simulink model "PIMPID"  (R2013b)
settings: Solver=FixedStepDiscrete  SolverMode=SingleTasking  StartTime=0.0  StopTime=100  FixedStep=0.1  RelTol=1e-3
libraries: xbsIndex_r4 x23, simulink x1
settings Model: Creator=laca  LastModifiedBy=laca

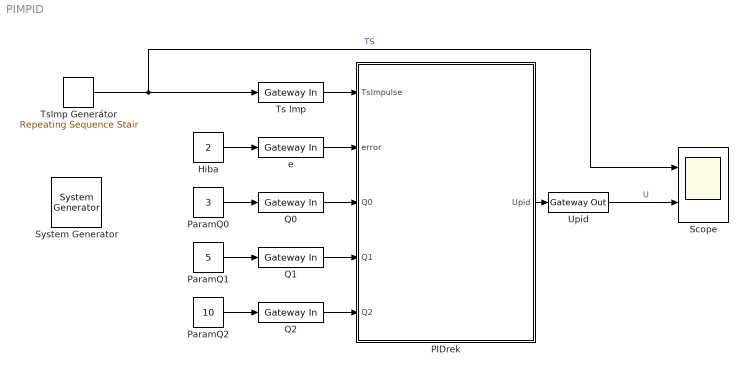
== system PIMPID ==
  " System Generator" : xbsIndex_r4/ System Generator  Tag=genX  xilinxfamily=spartan3e  part=xc3s500e  speed=-4  package=pq208  synthesis_tool=XST  clock_wrapper=Clock Enables  directory=./netlist  proj_type=Project Navigator  Synth_file=XST Defaults  Impl_file=ISE Defaults  testbench=off  simulink_period=1  sysclk_period=20  dcm_input_clock_period=10  incr_netlist=off  trim_vbits=Everywhere in SubSystem  dbl_ovrd=According to Block Masks  core_generation=According to Block Masks  run_coregen=off  deprecated_control=off  eval_field=0  block_type=sysgen
  Hiba : Constant  Value=2
  PIDrek : Subsystem
  ParamQ0 : Constant  Value=3
  ParamQ1 : Constant  Value=5
  ParamQ2 : Constant  Value=10
  Q0 : xbsIndex_r4/Gateway In  gui_display_data_type=Fixed-point  arith_type="Signed  (2's comp)"  n_bits=16  bin_pt=0  preci_type=Single  exp_width=8  frac_width=24  quantization="Round  (unbiased: +/- Inf)"  overflow=Saturate  period=1  dbl_ovrd=off  timing_constraint=None  locs_specified=off  LOCs={}  UseAsADC=off  ADCChannel='1'  inherit_from_input=off  hdl_port=on  block_type=gatewayin
  Q1 : xbsIndex_r4/Gateway In  gui_display_data_type=Fixed-point  arith_type="Signed  (2's comp)"  n_bits=16  bin_pt=0  preci_type=Single  exp_width=8  frac_width=24  quantization="Round  (unbiased: +/- Inf)"  overflow=Saturate  period=1  dbl_ovrd=off  timing_constraint=None  locs_specified=off  LOCs={}  UseAsADC=off  ADCChannel='1'  inherit_from_input=off  hdl_port=on  block_type=gatewayin
  Q2 : xbsIndex_r4/Gateway In  gui_display_data_type=Fixed-point  arith_type="Signed  (2's comp)"  n_bits=16  bin_pt=0  preci_type=Single  exp_width=8  frac_width=24  quantization="Round  (unbiased: +/- Inf)"  overflow=Saturate  period=1  dbl_ovrd=off  timing_constraint=None  locs_specified=off  LOCs={}  UseAsADC=off  ADCChannel='1'  inherit_from_input=off  hdl_port=on  block_type=gatewayin
  Scope : Scope  NumInputPorts=2
      settings: TimeRange=100  YMin=0~-5  YMax=1~5  SaveName=SC
  Ts Imp : xbsIndex_r4/Gateway In  gui_display_data_type=Boolean  arith_type=Boolean  n_bits=16  bin_pt=14  preci_type=Single  exp_width=8  frac_width=24  quantization="Round  (unbiased: +/- Inf)"  overflow=Saturate  period=1  dbl_ovrd=off  timing_constraint=None  locs_specified=off  LOCs={}  UseAsADC=off  ADCChannel='1'  inherit_from_input=off  hdl_port=on  block_type=gatewayin
  TsImp Generátor : simulink/Sources/Repeating Sequence Stair  OutValues="[0 0 1  0 0 0 0 0 0 0 0 0 0 0 0 0 0 0 0 0 ].'"  tsamp=1  OutMin=[]  OutMax=[]  OutDataTypeStr=fixdt('boolean')  OutputDataTypeScalingMode=Specify via dialog  OutDataType=fixdt('boolean')  ConRadixGroup=Best Precision: Vector-wise  OutScaling=[]
  Upid : xbsIndex_r4/Gateway Out  inherit_from_input=off  hdl_port=on  timing_constraint=None  locs_specified=off  LOCs={}  UseAsDAC=off  DACChannel='1'  block_type=gatewayout
  e : xbsIndex_r4/Gateway In  gui_display_data_type=Fixed-point  arith_type="Signed  (2's comp)"  n_bits=16  bin_pt=0  preci_type=Single  exp_width=8  frac_width=24  quantization="Round  (unbiased: +/- Inf)"  overflow=Saturate  period=1  dbl_ovrd=off  timing_constraint=None  locs_specified=off  LOCs={}  UseAsADC=off  ADCChannel='1'  inherit_from_input=off  hdl_port=on  block_type=gatewayin
  wires:
  Ts Imp/1 -> PIDrek/1(TsImpulse)
  Hiba/1 -> e/1
  ParamQ0/1 -> Q0/1
  ParamQ1/1 -> Q1/1
  ParamQ2/1 -> Q2/1
  Upid/1 -> Scope/2  "U"
  TsImp Generátor/1 -> Scope/1, Ts Imp/1  "TS"
  PIDrek/1(Upid) -> Upid/1
  e/1 -> PIDrek/2(error)
  Q0/1 -> PIDrek/3(Q0)
  Q1/1 -> PIDrek/4(Q1)
  Q2/1 -> PIDrek/5(Q2)

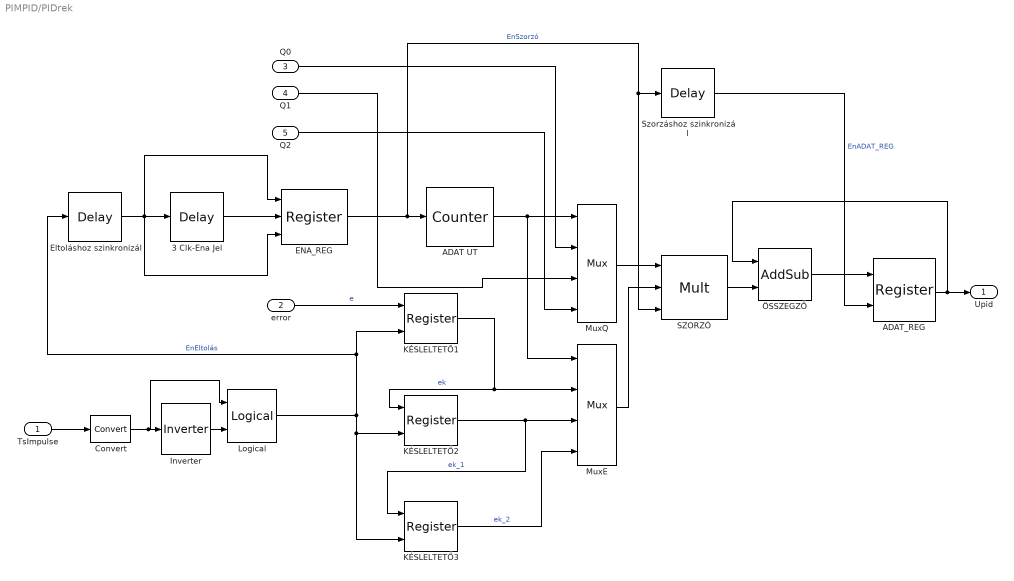
== system PIMPID/PIDrek ==
  TsImpulse : Inport
  error : Inport  Port=2
  Q0 : Inport  Port=3
  Q1 : Inport  Port=4
  Q2 : Inport  Port=5
  3 Clk-Ena Jel : xbsIndex_r4/Delay  rst=off  infoeditControl=Selection of Reset will increase slice count due to use of real FFs and instead of SRLs  en=off  latency=3  dbl_ovrd=off  reg_retiming=off  block_type=delay
  ADAT UT : xbsIndex_r4/Counter  cnt_type=Count Limited  cnt_to=2  operation=Up  start_count=0  cnt_by_val=1  arith_type=Unsigned  n_bits=2  bin_pt=0  load_pin=off  rst=off  en=on  explicit_period=on  period=1  dbl_ovrd=off  use_behavioral_HDL=off  implementation=Fabric  block_type=counter
      settings: xl_area=[100,0,0,0,0,0,0]
  ADAT_REG : xbsIndex_r4/Register  init=0  rst=off  en=on  dbl_ovrd=off  block_type=register
      settings: xl_area=[100,0,0,0,0,0,0]
  Convert : xbsIndex_r4/Convert  gui_display_data_type=Boolean  arith_type=Boolean  n_bits=16  bin_pt=14  float_type=Single  exp_bits=8  fraction_bits=24  quantization=Truncate  overflow=Wrap  en=off  latency=0  dbl_ovrd=off  pipeline=off  block_type=convert
  ENA_REG : xbsIndex_r4/Register  init=0  rst=on  en=on  dbl_ovrd=off  block_type=register
  Eltoláshoz szinkronizál : xbsIndex_r4/Delay  rst=off  infoeditControl=Selection of Reset will increase slice count due to use of real FFs and instead of SRLs  en=off  latency=1  dbl_ovrd=off  reg_retiming=off  block_type=delay
  Inverter : xbsIndex_r4/Inverter  en=off  latency=1  dbl_ovrd=off  block_type=inv
  KÉSLELTETŐ1 : xbsIndex_r4/Register  init=0  rst=off  en=on  dbl_ovrd=off  block_type=register
      settings: xl_area=[100,0,0,0,0,0,0]
  KÉSLELTETŐ2 : xbsIndex_r4/Register  init=0  rst=off  en=on  dbl_ovrd=off  block_type=register
      settings: xl_area=[100,0,0,0,0,0,0]
  KÉSLELTETŐ3 : xbsIndex_r4/Register  init=0  rst=off  en=on  dbl_ovrd=off  block_type=register
  Logical : xbsIndex_r4/Logical  logical_function=AND  inputs=2  en=off  latency=0  precision=Full  arith_type=Unsigned  n_bits=16  bin_pt=0  align_bp=on  dbl_ovrd=off  block_type=logical
  MuxE : xbsIndex_r4/Mux  inputs=3  en=off  latency=0  precision=User Defined  arith_type="Signed  (2's comp)"  n_bits=16  bin_pt=0  quantization=Truncate  overflow=Wrap  dbl_ovrd=off  block_type=mux
      settings: xl_use_area=on  xl_area=[1,0,0,0,0,0,0]
  MuxQ : xbsIndex_r4/Mux  inputs=3  en=off  latency=0  precision=User Defined  arith_type="Signed  (2's comp)"  n_bits=16  bin_pt=0  quantization=Truncate  overflow=Wrap  dbl_ovrd=off  block_type=mux
      settings: xl_area=[1,0,0,0,0,0,0]
  SZORZÓ : xbsIndex_r4/Mult  precision=User Defined  arith_type="Signed  (2's comp)"  n_bits=17  bin_pt=0  quantization=Truncate  overflow=Wrap  en=on  latency=1  dbl_ovrd=off  use_behavioral_HDL=off  opt=Area  use_embedded=on  optimum_pipeline=off  pipeline=on  use_rpm=on  placement_style=Triangular  block_type=mult
  Szorzáshoz szinkronizál : xbsIndex_r4/Delay  rst=off  infoeditControl=Selection of Reset will increase slice count due to use of real FFs and instead of SRLs  en=off  latency=1  dbl_ovrd=off  reg_retiming=off  block_type=delay
  ÖSSZEGZŐ : xbsIndex_r4/AddSub  mode=Addition  use_carryin=off  use_carryout=off  en=off  latency=0  precision=User Defined  arith_type="Signed  (2's comp)"  n_bits=17  bin_pt=0  quantization=Truncate  overflow=Saturate  dbl_ovrd=off  use_behavioral_HDL=off  hw_selection=Fabric  pipelined=off  block_type=addsub
      settings: xl_area=[100,0,0,0,0,0,0]
  Upid : Outport
  wires:
  MuxQ/1 -> SZORZÓ/1
  MuxE/1 -> SZORZÓ/2
  KÉSLELTETŐ2/1 -> KÉSLELTETŐ3/1, MuxE/3  "ek_1"
  ÖSSZEGZŐ/1 -> ADAT_REG/1
  3 Clk-Ena Jel/1 -> ENA_REG/2
  SZORZÓ/1 -> ÖSSZEGZŐ/2
  Szorzáshoz szinkronizál/1 -> ADAT_REG/2  "EnADAT_REG"
  ADAT_REG/1 -> Upid/1, ÖSSZEGZŐ/1
  ADAT UT/1 -> MuxE/1, MuxQ/1
  ENA_REG/1 -> Szorzáshoz szinkronizál/1, SZORZÓ/3, ADAT UT/1  "EnSzorzó"
  Q2/1 -> MuxQ/4
  KÉSLELTETŐ3/1 -> MuxE/4  "ek_2"
  Eltoláshoz szinkronizál/1 -> 3 Clk-Ena Jel/1, ENA_REG/3, ENA_REG/1
  KÉSLELTETŐ1/1 -> MuxE/2, KÉSLELTETŐ2/1  "ek"
  Q0/1 -> MuxQ/2
  Q1/1 -> MuxQ/3
  Inverter/1 -> Logical/2
  TsImpulse/1 -> Convert/1
  Logical/1 -> KÉSLELTETŐ3/2, KÉSLELTETŐ2/2, Eltoláshoz szinkronizál/1, KÉSLELTETŐ1/2  "EnEltolás"
  error/1 -> KÉSLELTETŐ1/1  "e"
  Convert/1 -> Inverter/1, Logical/1
